simulink model "flann_architecture"  (R2024b)
settings: Solver=FixedStepAuto  StartTime=0.0  StopTime=0.00016668  FixedStep=2.7777777777777777E-8  RelTol=1e-3
settings Model: Creator=HP  LastModifiedBy=HP

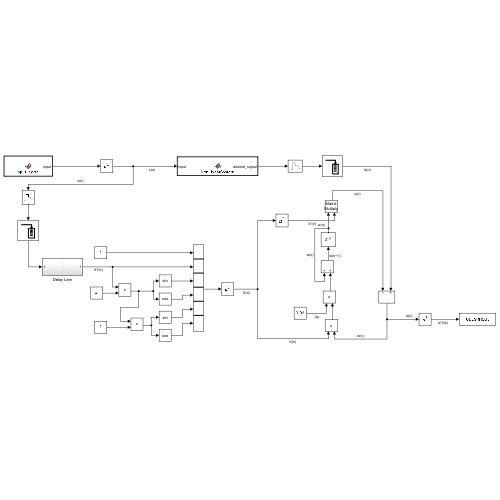
[thumbnail: Simulink's stored preview of the top-level diagram]
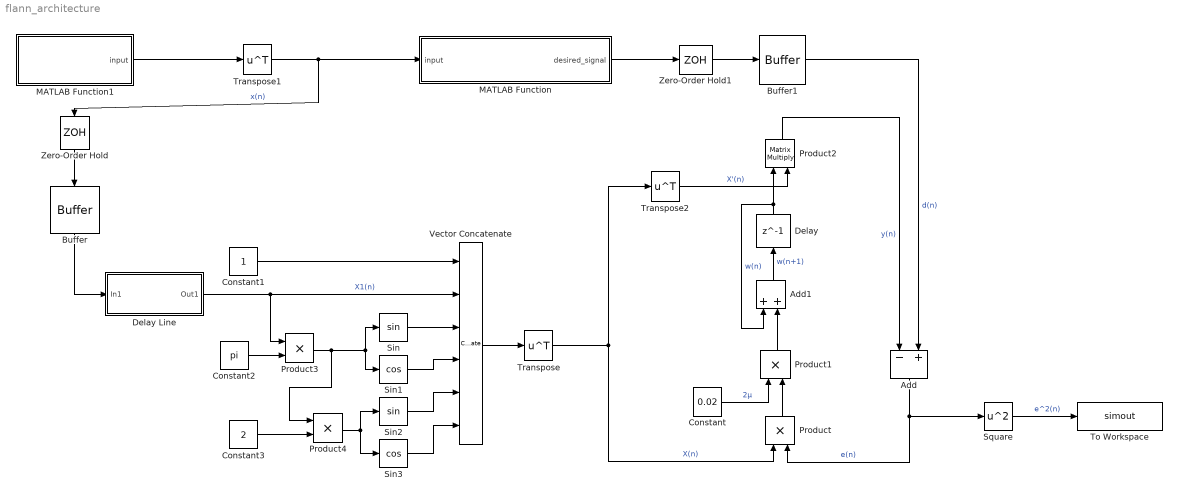
== system flann_architecture ==
  Add : Sum  Inputs=-+
  Add1 : Sum
  Buffer : Buffer  N=1  OutputFrames=off
  Buffer1 : Buffer  N=1  OutputFrames=off
  Constant : Constant  Value=0.02
  Constant1 : Constant
  Constant2 : Constant  Value=pi
  Constant3 : Constant  Value=2
  Delay : Delay  DelayLength=1  InputProcessing=Columns as channels (frame based)
  Delay Line : Subsystem
  MATLAB Function : MATLAB Function  TreatAsAtomicUnit=on
  MATLAB Function1 : MATLAB Function  TreatAsAtomicUnit=on
  Product{,1,3..4} (4 alike) : Product
  Product2 : Product  Multiplication=Matrix(*)
  Sin : Trigonometry
  Sin1 : Trigonometry  Operator=cos
  Sin2 : Trigonometry
  Sin3 : Trigonometry  Operator=cos
  Square : Math  Operator=square
  To Workspace : ToWorkspace  VariableName=simout  SaveFormat=Timeseries  SampleTime=-1
  Transpose : Math  Operator=transpose
  Transpose1 : Math  Operator=transpose
  Transpose2 : Math  Operator=transpose
  Vector Concatenate : Concatenate  NumInputs=6
  Zero-Order Hold : ZeroOrderHold  SampleTime=1/(6e3)
  Zero-Order Hold1 : ZeroOrderHold  SampleTime=1/(6e3)
  wires:
  Add/1 -> Square/1, Product/2  "e(n)"
  Product/1 -> Product1/2
  Constant/1 -> Product1/1  "2μ"
  Product1/1 -> Add1/2
  Add1/1 -> Delay/1  "w(n+1)"
  Product2/1 -> Add/1  "y(n)"
  Constant1/1 -> Vector Concatenate/1
  Delay Line/1(Out1) -> Vector Concatenate/2, Product3/1  "X1(n)"
  Product3/1 -> Sin/1, Sin1/1, Product4/1
  Sin/1 -> Vector Concatenate/3
  Constant2/1 -> Product3/2
  Sin1/1 -> Vector Concatenate/4
  Constant3/1 -> Product4/2
  Sin2/1 -> Vector Concatenate/5
  Product4/1 -> Sin2/1, Sin3/1
  Sin3/1 -> Vector Concatenate/6
  MATLAB Function1/1(input) -> Transpose1/1
  Transpose1/1 -> Zero-Order Hold/1, MATLAB Function/1(input)  "x(n)"
  Vector Concatenate/1 -> Transpose/1
  Buffer1/1 -> Add/2  "d(n)"
  MATLAB Function/1(desired_signal) -> Zero-Order Hold1/1
  Zero-Order Hold1/1 -> Buffer1/1
  Square/1 -> To Workspace/1  "e^2(n)"
  Buffer/1 -> Delay Line/1(In1)
  Transpose/1 -> Transpose2/1, Product/1  "X(n)"
  Transpose2/1 -> Product2/2  "X'(n)"
  Zero-Order Hold/1 -> Buffer/1
  Delay/1 -> Add1/1, Product2/1  "w(n)"

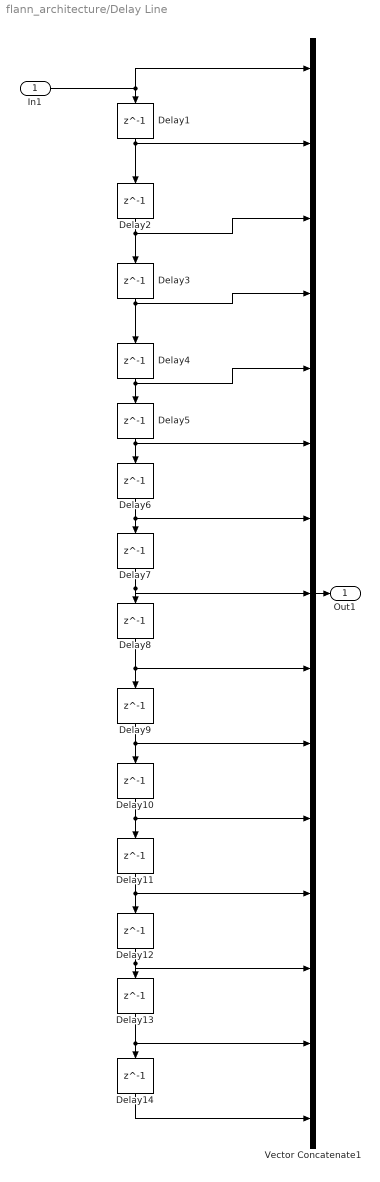
== system flann_architecture/Delay Line ==
  In1 : Inport
  Delay{1..14} (14 alike) : Delay  DelayLength=1  InputProcessing=Columns as channels (frame based)
  Vector Concatenate1 : Concatenate  NumInputs=15
  Out1 : Outport
  wires:
  Delay14/1 -> Vector Concatenate1/15
  Delay5/1 -> Delay6/1, Vector Concatenate1/6
  Delay6/1 -> Delay7/1, Vector Concatenate1/7
  Delay3/1 -> Delay4/1, Vector Concatenate1/4
  Delay8/1 -> Delay9/1, Vector Concatenate1/9
  Delay12/1 -> Vector Concatenate1/13, Delay13/1
  In1/1 -> Delay1/1, Vector Concatenate1/1
  Delay13/1 -> Vector Concatenate1/14, Delay14/1
  Delay7/1 -> Delay8/1, Vector Concatenate1/8
  Delay11/1 -> Vector Concatenate1/12, Delay12/1
  Delay2/1 -> Delay3/1, Vector Concatenate1/3
  Delay9/1 -> Delay10/1, Vector Concatenate1/10
  Delay4/1 -> Vector Concatenate1/5, Delay5/1
  Delay1/1 -> Delay2/1, Vector Concatenate1/2
  Delay10/1 -> Delay11/1, Vector Concatenate1/11
  Vector Concatenate1/1 -> Out1/1

== matlab function flann_architecture/MATLAB Function ==
  data: input input; desired_signal output
function desired_signal = NonLinearSystem(input)
    % Preallocate the output vector for efficiency
    desired_signal = zeros(size(input));
    
    % Compute the noise for the entire input
    noise = awgn(input, 30) - input;
    
    for i = 1:length(input)
        % Compute the nonlinear operation for input(i)
        q = 1.5 * input(i) - 0.3 * input(i)^2 ;
        
        % Choose the parameter 'rho' based on the sign of q
        if q > 0
            rho = 4;
        else
            rho = 0.5;
        end
        
        % Compute the desired signal for element i
        desired_signal(i) = 2 * ((1/(1+exp(-rho*q)))-0.5) + noise(i);
    end
end

== matlab function flann_architecture/MATLAB Function1 ==
  data: input output
function input = input_signal()

    rng('shuffle'); % Ensures different random numbers each run
    no_of_inputs = 6e3;
    input = rand(1, no_of_inputs) - 0.5; % Range: [-0.5, 0.5]
end
